simulink model "costas_ClosedLoop"  (Simulink 7.6)
settings: Solver=ode45  StartTime=0.0  StopTime=16  RelTol=1e-3
libraries: dsparch4 x3, commsynccomp2 x2, commseqgen2 x1, commutil2 x1
Description:
  | Costas Loop for PSK Closedloop
  | (C)McCrocodile ZHENG 2010.8.18
settings Model: Creator=McCrocodile  LastModifiedBy=McCrocodile

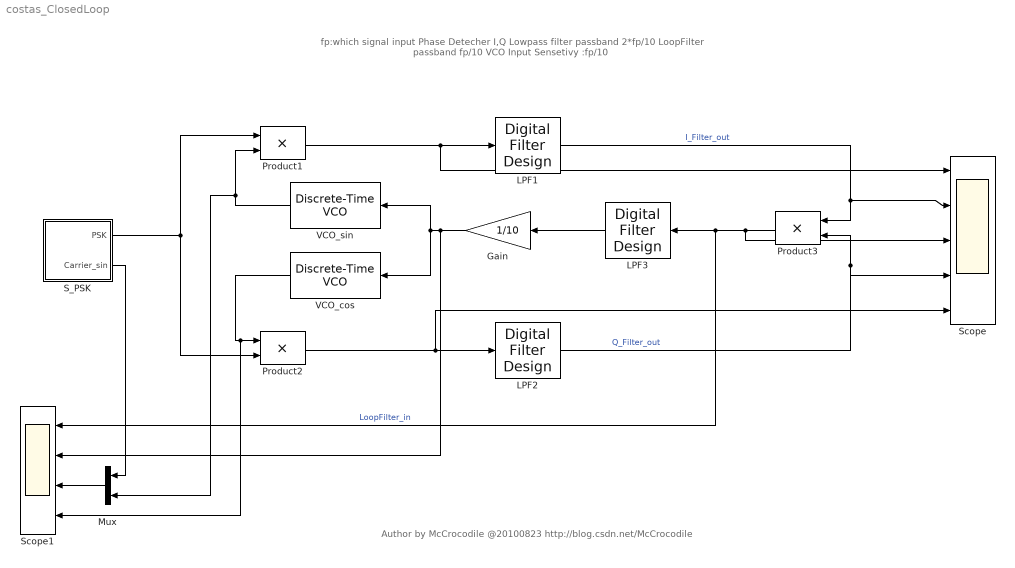
== system costas_ClosedLoop ==
  note: Author by McCrocodile  @20100823
      | http://blog.csdn.net/McCrocodile
  note: fp:which signal input Phase Detecher
      | I,Q Lowpass filter passband 2*fp/10
      | LoopFilter passband fp/10
      | VCO Input Sensetivy :fp/10
  Gain : Gain  Gain=1/10
  LPF1 : dsparch4/Digital Filter Design  SystemSampleTime=-1  mwdsp_browser_bugfix_var=off
  LPF2 : dsparch4/Digital Filter Design  SystemSampleTime=-1  mwdsp_browser_bugfix_var=off
  LPF3 : dsparch4/Digital Filter Design  SystemSampleTime=-1  mwdsp_browser_bugfix_var=off
  Mux : Mux  Inputs=2
  Product1 : Product  SaturateOnIntegerOverflow=on  OutDataTypeStr=Inherit: Same as first input
  Product2 : Product  SaturateOnIntegerOverflow=on  OutDataTypeStr=Inherit: Same as first input
  Product3 : Product  SaturateOnIntegerOverflow=on  OutDataTypeStr=Inherit: Same as first input
  S_PSK : Subsystem
  Scope : Scope  NumInputPorts=5
      settings: TimeRange=0.5  YMin=-1~-0.75~-0.15~-0.75~-1  YMax=1~0.75~0.15~0.75~1  MaxDataPoints=50000
  Scope1 : Scope  NumInputPorts=4
      settings: TimeRange=0.6000000000000001  YMin=-0.01~-7.5e-005~-1.25~-1  YMax=0.0075~7.5e-005~1.25~1  MaxDataPoints=50000
  VCO_cos : commsynccomp2/Discrete-Time VCO  SystemSampleTime=-1  Ac=1  Fc=10.7e3  Kc=1e3  Ph=pi/2  ts=1e-5
  VCO_sin : commsynccomp2/Discrete-Time VCO  SystemSampleTime=-1  Ac=1  Fc=10.7e3  Kc=1e3  Ph=0  ts=1e-5
  wires:
  S_PSK/1(PSK) -> Product1/1, Product2/2
  VCO_cos/1 -> Product2/1, Scope1/4
  Product1/1 -> LPF1/1, Scope/1
  Product2/1 -> Scope/5, LPF2/1
  LPF1/1 -> Product3/1, Scope/2  "I_Filter_out"
  LPF2/1 -> Product3/2, Scope/4  "Q_Filter_out"
  Product3/1 -> Scope/3, Scope1/1, LPF3/1  "LoopFilter_in"
  VCO_sin/1 -> Product1/2, Mux/2
  Mux/1 -> Scope1/3
  S_PSK/2(Carrier_sin) -> Mux/1
  Gain/1 -> VCO_sin/1, VCO_cos/1, Scope1/2
  LPF3/1 -> Gain/1

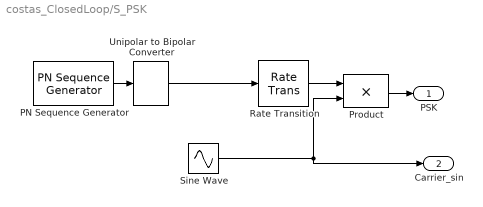
== system costas_ClosedLoop/S_PSK ==
  PN Sequence Generator : commseqgen2/PN Sequence Generator  poly=[1 0 0 0 0 1 1]  ini_sta=[0 0 0 0 0 1]  outBitMaskSource=Dialog parameter  shift=0  Ts=1/32  frameBased=off  sampPerFrame=1  reset=off  bitPackedOutputs=off  outDataType=double  numPackedBits=8  bitPackDataSigned=off  bitPackedOutDType=double
  Product : Product  SaturateOnIntegerOverflow=on  OutDataTypeStr=Inherit: Same as first input
  Rate Transition : RateTransition
  Sine Wave : Sin  Frequency=10.7e3*2*pi  Phase=pi/2  SampleTime=1e-5
  Unipolar to Bipolar Converter : commutil2/Unipolar to Bipolar Converter  SystemSampleTime=-1  M=2  polarity=Positive  dataType=Same as input
  PSK : Outport
  Carrier_sin : Outport  Port=2
  wires:
  PN Sequence Generator/1 -> Unipolar to Bipolar Converter/1
  Rate Transition/1 -> Product/1
  Sine Wave/1 -> Product/2, Carrier_sin/1
  Product/1 -> PSK/1
  Unipolar to Bipolar Converter/1 -> Rate Transition/1
